simulink model "deltino"  (R2021b)
settings: Solver=VariableStepAuto  StartTime=0.0  StopTime=inf  FixedStep=0.0001  RelTol=1e-3
values from neighbouring files (symbols this model uses):
  alpha1 = 0    [compute_deltino_dyn_parallel.m]
  alpha2 = 2/3*pi    (= 2.09439510239)    [compute_deltino_dyn_parallel.m]
  alpha3 = 4/3*pi    (= 4.18879020479)    [compute_deltino_dyn_parallel.m]
  H = 0.05    [main.m]
  J_T = [J_1', J_2', J_3', J_4']    [main.m]
  K_d = 10    [main.m]
  K_el = 10000    [main.m]
  K_i = 1    [main.m]
  K_p = 200    [main.m]
  K_v = 10    [main.m]
  mu = 0.8    [main.m]
  ni_0 = zeros(18,1)    [main.m]
  offset1 = [l1/2; l2/2; -h/2]    [compute_deltino_dyn_parallel.m]    (also in main.m = [+l1/2; +l2/2; -h/2])
  offset2 = [l1/2; -l2/2; -h/2]    [compute_deltino_dyn_parallel.m]    (also in main.m = [+l1/2; -l2/2; -h/2])
  offset3 = [-l1/2; -l2/2; -h/2]    [compute_deltino_dyn_parallel.m]    (also in main.m)
  offset4 = [-l1/2; l2/2; -h/2]    [compute_deltino_dyn_parallel.m]    (also in main.m = [-l1/2; +l2/2; -h/2])
  p_leg1_0 = forward_kin(theta_leg1_0)    [main.m]
  p_leg2_0 = forward_kin(theta_leg2_0)    [main.m]
  p_leg3_0 = forward_kin(theta_leg3_0)    [main.m]
  p_leg4_0 = forward_kin(theta_leg4_0)    [main.m]
  points_ccw = [+0.1,  0.00 ... (first row only)    [main.m]
  points_cw = [-0.1,  0.00 ... (first row only)    [main.m]
  q_0 = [base_0; ypr_0; theta_leg1_0; ee_leg1_0; theta_leg2_0; ee_leg2_0;        theta_leg3_0; ee_leg3_0; theta_leg4_0; ee_leg4_0;]    [main.m]
  ratio = 2    [main.m]
  steps = 4+2*ratio    (= 8)    [main.m]
  theta_leg1_0 = [pi/6; pi/6; pi/6]    [main.m]
  theta_leg2_0 = [pi/6; pi/6; pi/6]    [main.m]
  theta_leg3_0 = [pi/6; pi/6; pi/6]    [main.m]
  theta_leg4_0 = [pi/6; pi/6; pi/6]    [main.m]
  ts = T/steps    (= 0.1875)    [main.m]
  ts2 = 3*ts    (= 0.5625)    [main.m]
  vel = 0.2    [main.m]
undefined symbols (not defined in the file or in its folder): l1, l_A, l_B, R, radius0, radius1, radius2, theta, WPs
libraries: simulink x14, dspsigops x12
(part 10 of 10)

== matlab function deltino/DELTINO DYNAMICS /compute_G ==
  data: q input; G output
function G = G(q)
%#codegen

%    This function was generated by the Symbolic Math Toolbox version 9.0.
%    03-May-2022 23:38:54
zeta = q(5); psi = q(6);
th11 = q(7); th12 = q(8); th13 = q(9);
th21 = q(13); th22 = q(14); th23 = q(15);
th31 = q(19); th32 = q(20); th33 = q(21);
th41 = q(25); th42 = q(26); th43 = q(27);
t2 = cos(psi);
t3 = cos(th11);
t4 = cos(th12);
t5 = cos(th13);
t6 = cos(th21);
t7 = cos(th22);
t8 = cos(th23);
t9 = cos(th31);
t10 = cos(th32);
t11 = cos(th33);
t12 = cos(th41);
t13 = cos(th42);
t14 = cos(th43);
t15 = cos(zeta);
t16 = sin(psi);
t17 = sin(th11);
t18 = sin(th12);
t19 = sin(th13);
t20 = sin(th21);
t21 = sin(th22);
t22 = sin(th23);
t23 = sin(th31);
t24 = sin(th32);
t25 = sin(th33);
t26 = sin(th41);
t27 = sin(th42);
t28 = sin(th43);
t29 = sin(zeta);
t30 = sqrt(3.0);
t31 = t15./2.0;
t32 = t29./2.0;
t35 = t15.*t16.*t30.*(-1.0./2.0);
t36 = t16.*t29.*t30.*(-1.0./2.0);
t33 = t16.*t30.*t31;
t34 = t16.*t30.*t32;
t39 = t31+t36;
t40 = t32+t35;
t37 = t31+t34;
t38 = t32+t33;
et1 = t15.*(-2.94e+2./1.25e+2)+t37.*(t5.*(3.0./2.0e+1)+3.0./2.0e+1).*(9.8e+1./2.5e+1)+t39.*(t4.*(3.0./2.0e+1)+3.0./2.0e+1).*(9.8e+1./2.5e+1)+t37.*(t8.*(3.0./2.0e+1)+3.0./2.0e+1).*(9.8e+1./2.5e+1)+t39.*(t7.*(3.0./2.0e+1)+3.0./2.0e+1).*(9.8e+1./2.5e+1)+t37.*(t11.*(3.0./2.0e+1)+3.0./2.0e+1).*(9.8e+1./2.5e+1)+t39.*(t10.*(3.0./2.0e+1)+3.0./2.0e+1).*(9.8e+1./2.5e+1)+t37.*(t14.*(3.0./2.0e+1)+3.0./2.0e+1).*(9.8e+1./2.5e+1)+t39.*(t13.*(3.0./2.0e+1)+3.0./2.0e+1).*(9.8e+1./2.5e+1)-t3.*t15.*(1.47e+2./2.5e+2)-t6.*t15.*(1.47e+2./2.5e+2)-t9.*t15.*(1.47e+2./2.5e+2);
et2 = t12.*t15.*(-1.47e+2./2.5e+2)+t2.*t29.*(5.88e+2./1.25e+2)+t2.*t17.*t29.*(1.47e+2./2.5e+2)+t2.*t18.*t29.*(1.47e+2./2.5e+2)+t2.*t19.*t29.*(1.47e+2./2.5e+2)+t2.*t20.*t29.*(1.47e+2./2.5e+2)+t2.*t21.*t29.*(1.47e+2./2.5e+2)+t2.*t22.*t29.*(1.47e+2./2.5e+2)+t2.*t23.*t29.*(1.47e+2./2.5e+2)+t2.*t24.*t29.*(1.47e+2./2.5e+2)+t2.*t25.*t29.*(1.47e+2./2.5e+2)+t2.*t26.*t29.*(1.47e+2./2.5e+2)+t2.*t27.*t29.*(1.47e+2./2.5e+2)+t2.*t28.*t29.*(1.47e+2./2.5e+2);
mt1 = [0.0;0.0;7.644e+1;0.0;et1+et2;t15.*(t16.*1.6e+1+t16.*t17.*2.0+t16.*t18.*2.0+t16.*t19.*2.0+t16.*t20.*2.0+t16.*t21.*2.0+t16.*t22.*2.0+t16.*t23.*2.0+t16.*t24.*2.0+t16.*t25.*2.0+t16.*t26.*2.0+t16.*t27.*2.0+t16.*t28.*2.0+t2.*t4.*t30-t2.*t5.*t30+t2.*t7.*t30-t2.*t8.*t30+t2.*t10.*t30-t2.*t11.*t30+t2.*t13.*t30-t2.*t14.*t30).*(1.47e+2./5.0e+2);t17.*t29.*(1.47e+2./2.5e+2)-t2.*t3.*t15.*(1.47e+2./2.5e+2);t18.*t38.*(-1.47e+2./2.5e+2)-t2.*t4.*t15.*(1.47e+2./2.5e+2);t19.*t40.*(-1.47e+2./2.5e+2)-t2.*t5.*t15.*(1.47e+2./2.5e+2);0.0;0.0;4.41e+2./1.0e+2];
mt2 = [t20.*t29.*(1.47e+2./2.5e+2)-t2.*t6.*t15.*(1.47e+2./2.5e+2);t21.*t38.*(-1.47e+2./2.5e+2)-t2.*t7.*t15.*(1.47e+2./2.5e+2);t22.*t40.*(-1.47e+2./2.5e+2)-t2.*t8.*t15.*(1.47e+2./2.5e+2);0.0;0.0;4.41e+2./1.0e+2;t23.*t29.*(1.47e+2./2.5e+2)-t2.*t9.*t15.*(1.47e+2./2.5e+2);t24.*t38.*(-1.47e+2./2.5e+2)-t2.*t10.*t15.*(1.47e+2./2.5e+2);t25.*t40.*(-1.47e+2./2.5e+2)-t2.*t11.*t15.*(1.47e+2./2.5e+2);0.0;0.0;4.41e+2./1.0e+2;t26.*t29.*(1.47e+2./2.5e+2)-t2.*t12.*t15.*(1.47e+2./2.5e+2)];
mt3 = [t27.*t38.*(-1.47e+2./2.5e+2)-t2.*t13.*t15.*(1.47e+2./2.5e+2);t28.*t40.*(-1.47e+2./2.5e+2)-t2.*t14.*t15.*(1.47e+2./2.5e+2);0.0;0.0;4.41e+2./1.0e+2];
G = [mt1;mt2;mt3];
